simulink model "c2f_twochannel"  (R2019b)
settings: Solver=ode45  StartTime=0.0  StopTime=364  RelTol=1e-3  EnableMultiTasking=on
PreLoadFcn:
  | t = [0:364]';
  | load bangaloreTempsC
  | T = [TmaxC,TminC];
StopFcn:
  | plot(tout,yout); grid on;
  | xlabel('Day of the year');
  | ylabel('Temperature ( ^oF)');
  | title('Bangalore Daily Max and Min temperatures');
  | legend('Max Temp','Min Temp');
values from neighbouring files (symbols this model uses):
  TmaxC = [27.1111111111 27.7777777778 29.1111111111 30.2777777778 28.2222222222 29.1111111111 28.8888888889 26.7777777778 25.8888888889 30.2777777778 31.7777777778 30.5 ... (365 elements, 365x1)]    [bangaloreTempsC.mat]
  TminC = [18.3888888889 17.2777777778 17.6111111111 17.7777777778 15.8888888889 15.7222222222 14 15.8888888889 14.8888888889 13.8888888889 14.5 15.5 ... (365 elements, 365x1)]    [bangaloreTempsC.mat]
settings Model: Creator=bbhattac  LastModifiedBy=khung
settings DataIOCC: ExternalInput=[t, T]  LimitDataPoints=on  LoadExternalInput=on  SaveFormat=Array  SignalLoggingSaveFormat=ModelDataLogs  ReturnWorkspaceOutputs=off
settings OptimizationCC: ExpressionDepthLimit=2147483647  LifeSpan=inf
settings DebuggingCC: UnderspecifiedInitializationDetection=Classic  MergeDetectMultiDrivingBlocksExec=none  SolverPrmCheckMsg=warning  FcnCallInpInsideContextMsg=warning  StateNameClashWarn=warning  SFUnexpectedBacktrackingDiag=warning  SFNoUnconditionalDefaultTransitionDiag=warning  SFExecutionAtInitializationDiag=none  ArithmeticOperatorsInVariantConditions=warning
settings HardwareCC: ProdBitPerPointer=32  ProdBitPerSizeT=32  ProdBitPerPtrDiffT=32  ProdLargestAtomicFloat=None  ProdIntDivRoundTo=Undefined  ProdEndianess=Unspecified  ProdWordSize=32  ProdHWDeviceType=32-bit Generic
settings ModelReferenceCC: PropagateSignalLabelsOutOfModel=off
settings SFSimCC: SimUseLocalCustomCode=off
settings RTWCC: RTWUseLocalCustomCode=off
settings CodeAppCC: StateflowObjectComments=on
settings GRTTargetCC: TargetLangStandard=C89/C90 (ANSI)  GeneratePreprocessorConditionals=Disable all  CombineOutputUpdateFcns=off  GRTInterface=on
settings ConfigComp: CovMetricSettings=dw  CovHtmlReporting=on  CovSaveCumulativeToWorkspaceVar=on  CovSaveSingleToWorkspaceVar=on  CovExternalEMLEnable=off

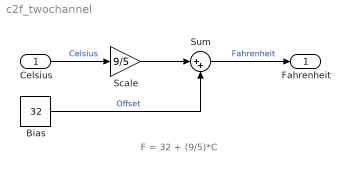
== system c2f_twochannel ==
  note: F = 32 + (9/5)*C
  Celsius : Inport  PortDimensions=2
  Bias : Constant  Value=32
  Scale : Gain  Gain=9/5
  Sum : Sum  Inputs=|++
  Fahrenheit : Outport
  wires:
  Celsius/1 -> Scale/1  "Celsius"
  Scale/1 -> Sum/1
  Bias/1 -> Sum/2  "Offset"
  Sum/1 -> Fahrenheit/1  "Fahrenheit"
